simulink model "P5"  (R2024a)
settings: Solver=ode45  StartTime=0.0  StopTime=5  RelTol=1e-3
settings Model: Creator=ahmad  LastModifiedBy=ahmad

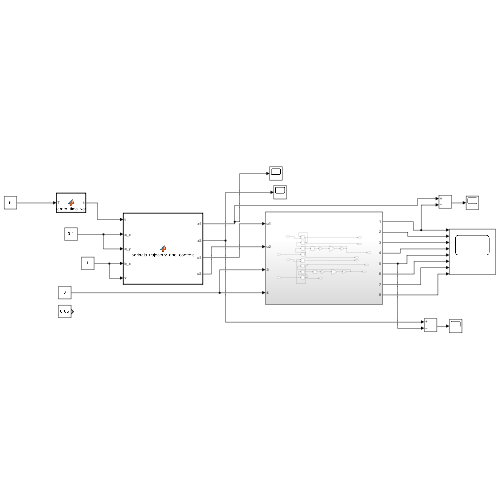
[thumbnail: Simulink's stored preview of the top-level diagram]
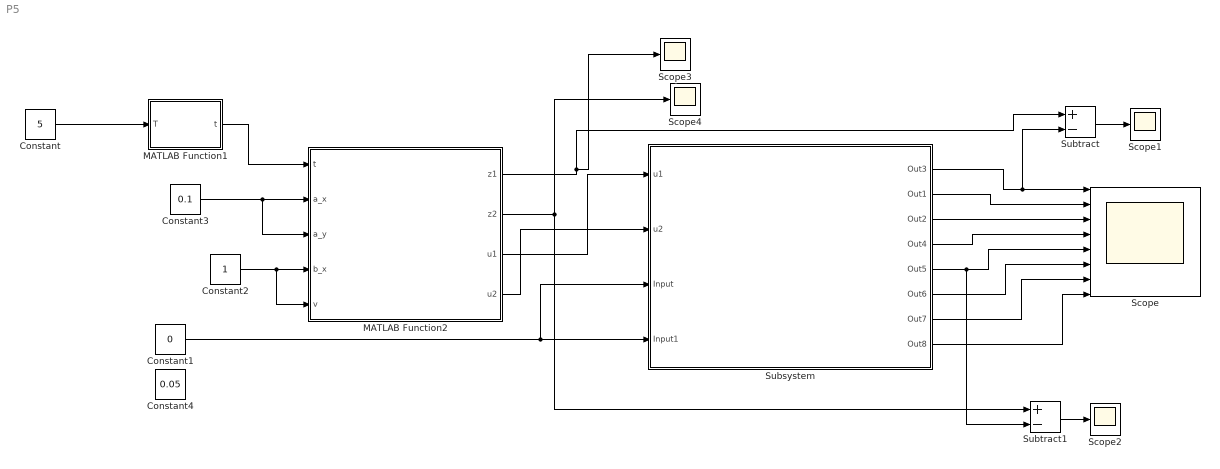
== system P5 ==
  Constant : Constant  Value=5
  Constant1 : Constant  Value=0
  Constant2 : Constant
  Constant3 : Constant  Value=0.1
  Constant4 : Constant  Value=0.05
  MATLAB Function1 : MATLAB Function  TreatAsAtomicUnit=on
  MATLAB Function2 : MATLAB Function  TreatAsAtomicUnit=on
  Scope : Scope  NumInputPorts=8
  Scope{1..4} (4 alike) : Scope
  Subsystem : Subsystem
  Subtract : Sum  Inputs=+-
  Subtract1 : Sum  Inputs=+-
  wires:
  MATLAB Function2/3(u1) -> Subsystem/1(u1)
  MATLAB Function2/4(u2) -> Subsystem/2(u2)
  Constant/1 -> MATLAB Function1/1(T)
  Constant1/1 -> Subsystem/4(Input1), Subsystem/3(Input)
  MATLAB Function1/1(t) -> MATLAB Function2/1(t)
  MATLAB Function2/1(z1) -> Scope3/1, Subtract/1
  MATLAB Function2/2(z2) -> Scope4/1, Subtract1/1
  Subsystem/1(Out3) -> Subtract/2, Scope/1
  Subsystem/2(Out1) -> Scope/2
  Subsystem/3(Out2) -> Scope/3
  Subsystem/4(Out4) -> Scope/4
  Subsystem/5(Out5) -> Subtract1/2, Scope/5
  Subsystem/6(Out6) -> Scope/6
  Subsystem/7(Out7) -> Scope/7
  Subsystem/8(Out8) -> Scope/8
  Subtract/1 -> Scope1/1
  Subtract1/1 -> Scope2/1
  Constant3/1 -> MATLAB Function2/3(a_y), MATLAB Function2/2(a_x)
  Constant2/1 -> MATLAB Function2/5(v), MATLAB Function2/4(b_x)

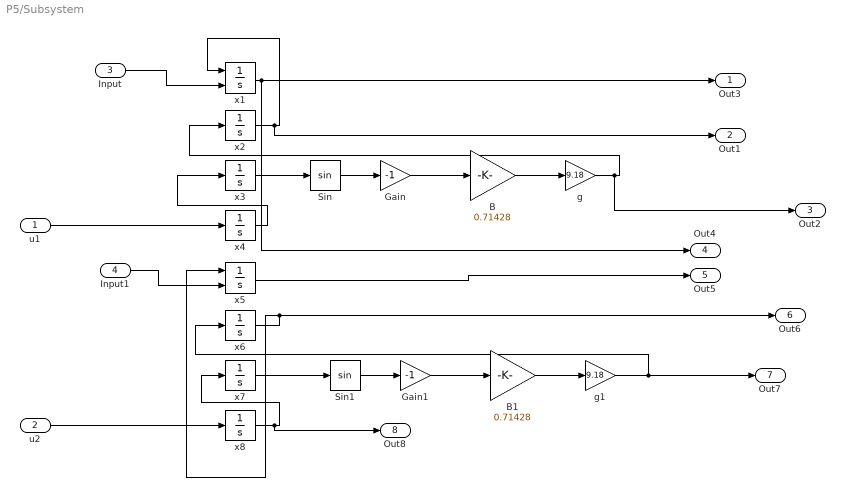
== system P5/Subsystem ==
  u1 : Inport
  u2 : Inport  Port=2
  Input : Inport  Port=3
  Input1 : Inport  Port=4
  B : Gain  Gain=0.71428
  B1 : Gain  Gain=0.71428
  Gain : Gain  Gain=-1
  Gain1 : Gain  Gain=-1
  Sin : Trigonometry
  Sin1 : Trigonometry
  g : Gain  Gain=9.18
  g1 : Gain  Gain=9.18
  x1 : Integrator  InitialConditionSource=external
  x{2..4,6..8} (6 alike) : Integrator
  x5 : Integrator  InitialConditionSource=external
  Out3 : Outport
  Out1 : Outport  Port=2
  Out2 : Outport  Port=3
  Out4 : Outport  Port=4
  Out5 : Outport  Port=5
  Out6 : Outport  Port=6
  Out7 : Outport  Port=7
  Out8 : Outport  Port=8
  wires:
  x2/1 -> Out1/1, x1/1
  B1/1 -> g1/1
  Gain1/1 -> B1/1
  x6/1 -> x5/1, Out6/1
  g/1 -> Out2/1, x2/1
  Sin1/1 -> Gain1/1
  B/1 -> g/1
  x8/1 -> Out8/1, x7/1
  x4/1 -> x3/1
  x3/1 -> Sin/1
  Gain/1 -> B/1
  x7/1 -> Sin1/1
  g1/1 -> x6/1, Out7/1
  x5/1 -> Out5/1
  Sin/1 -> Gain/1
  x1/1 -> Out4/1, Out3/1
  u2/1 -> x8/1
  u1/1 -> x4/1
  Input/1 -> x1/2
  Input1/1 -> x5/2

== matlab function P5/MATLAB Function1 ==
  data: T input; t output
function t = generate_time_vector(T)
    % Inputs: T is the total time
    % Outputs: t is a time vector
    t = linspace(0, T, 100);
end

== matlab function P5/MATLAB Function2 ==
  data: t input; z1 output; a_x input; a_y input; b_x input; v input; z2 output; u1 output; u2 output
function [z1, z2, u1, u2] = periodic_trajectory_and_controls(t, a_x, a_y, b_x, v)
% PERIODIC_TRAJECTORY_AND_CONTROLS Computes periodic desired trajectories and controls
% for the ball-on-plate system for both x- and y-directions.
%
% Inputs:
%   t     - Time variable (scalar or vector)
%   a_x   - Amplitude in x-direction
%   a_y   - Amplitude in y-direction
%   b_x   - Parameter defining the trajectory type (1 = circle, 2 = eight, 4 = double eight)
%   v     - Angular velocity (rad/s)
%
% Outputs:
%   z1    - Desired trajectory for x-direction
%   z2    - Desired trajectory for y-direction
%   u1    - Control input for x-direction (fourth derivative of z1)
%   u2    - Control input for y-direction (fourth derivative of z2)

    % Desired trajectory in x-direction (z1)
    z1 = a_x * sin(b_x * v * t);
    % Desired trajectory in y-direction (z2)
    z2 = a_y * cos(v * t);

    % First derivatives
    dz1 = a_x * b_x * v * cos(b_x * v * t);
    dz2 = -a_y * v * sin(v * t);

    % Second derivatives
    ddz1 = -a_x * b_x^2 * v^2 * sin(b_x * v * t);
    ddz2 = -a_y * v^2 * cos(v * t);

    % Third derivatives
    dddz1 = -a_x * b_x^3 * v^3 * cos(b_x * v * t);
    dddz2 = a_y * v^3 * sin(v * t);

    % Fourth derivatives (controls)
    u1 = a_x * b_x^4 * v^4 * sin(b_x * v * t);
    u2 = a_y * v^4 * cos(v * t);

end
